simulink model "harmonic"  (R2018b)
settings: Solver=FixedStepAuto  StartTime=0.0  StopTime=t  FixedStep=0.001  RelTol=1e-3
values from neighbouring files (symbols this model uses):
  freq = 10    [frekvencne.m]
settings Model: Creator=jakub  LastModifiedBy=jakub

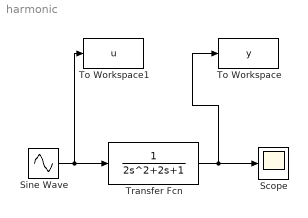
== system harmonic ==
  Scope : Scope
  Sine Wave : Sin  Frequency=freq  SampleTime=0
  To Workspace : ToWorkspace  VariableName=y  SaveFormat=Timeseries  SampleTime=-1
  To Workspace1 : ToWorkspace  VariableName=u  SaveFormat=Timeseries  SampleTime=-1
  Transfer Fcn : TransferFcn  Denominator=[2 2 1]
  wires:
  Transfer Fcn/1 -> To Workspace/1, Scope/1
  Sine Wave/1 -> To Workspace1/1, Transfer Fcn/1
